simulink model "pid_controller"  (R2017a)
settings: Solver=ode4  StartTime=0.0  StopTime=8  FixedStep=10^-3  RelTol=1e-3
settings Model: Creator=Sean  LastModifiedBy=Sean

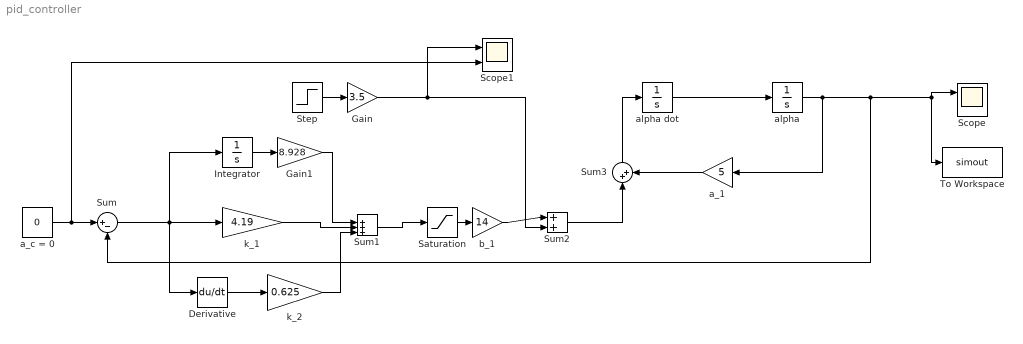
== system pid_controller ==
  Derivative : Derivative
  Gain : Gain  Gain=3.5
  Gain1 : Gain  Gain=8.928
  Integrator : Integrator
  Saturation : Saturate  UpperLimit=pi/3  LowerLimit=-pi/3
  Scope : Scope  NumInputPorts=2
  Scope1 : Scope  NumInputPorts=2
  Step : Step  Time=5  SampleTime=0
  Sum : Sum  Inputs=|+-
  Sum1 : Sum  Inputs=+|++
  Sum2 : Sum  Inputs=|++
  Sum3 : Sum  Inputs=|++
  To Workspace : ToWorkspace  VariableName=simout  SaveFormat=Timeseries  SampleTime=-1
  a_1 : Gain  Gain=5
  a_c = 0 : Constant  Value=0
  alpha : Integrator  InitialCondition=0.12
  alpha dot : Integrator  InitialCondition=0.45
  b_1 : Gain  Gain=14
  k_1 : Gain  Gain=4.19
  k_2 : Gain  Gain=0.625
  wires:
  b_1/1 -> Sum2/1
  Derivative/1 -> k_2/1
  k_2/1 -> Sum1/3
  Sum3/1 -> alpha dot/1
  a_1/1 -> Sum3/2
  k_1/1 -> Sum1/2
  Gain/1 -> Scope1/1, Sum2/2
  Sum2/1 -> Sum3/1
  Saturation/1 -> b_1/1
  Sum/1 -> Integrator/1, Derivative/1, k_1/1
  Sum1/1 -> Saturation/1
  alpha dot/1 -> alpha/1
  a_c = 0/1 -> Scope1/2, Sum/1
  Step/1 -> Gain/1
  Integrator/1 -> Gain1/1
  Gain1/1 -> Sum1/1
  alpha/1 -> Sum/2, To Workspace/1, Scope/1, a_1/1
